simulink model "TestHiTechnicColorSensor"  (Simulink 6.4)
settings: Solver=FixedStepDiscrete  SolverMode=SingleTasking  StartTime=0  StopTime=inf  FixedStep=0.001  RelTol=1e-3
libraries: simulink x9, ecrobot_nxt_lib x8
settings Model: Creator=tchikama  LastModifiedBy=tchikama  ProdHWDeviceType=ARM7
settings DataIOCC: SaveOutput=off  SignalLogging=off  SaveTime=off
settings OptimizationCC: InlineParams=on  InlineInvariantSignals=on  RollThreshold=2  StateBitsets=on  DataBitsets=on  UseTempVars=on  InitFltsAndDblsToZero=off  NoFixptDivByZeroProtection=on  EfficientFloat2IntCast=on  OptimizeModelRefInitCode=on  LifeSpan=1
settings DebuggingCC: ConsistencyChecking=warning  SignalInfNanChecking=warning  ReadBeforeWriteMsg=DisableAll  WriteAfterWriteMsg=DisableAll  WriteAfterReadMsg=DisableAll  AlgebraicLoopMsg=error  CheckExecutionContextPreStartOutputMsg=on  CheckExecutionContextRuntimeOutputMsg=on  SolverPrmCheckMsg=none  SingleTaskRateTransMsg=warning  TasksWithSamePriorityMsg=none  IntegerOverflowMsg=error  ParameterPrecisionLossMsg=none  UnconnectedInputMsg=error  UnconnectedOutputMsg=error  UnconnectedLineMsg=error  UniqueDataStoreMsg=error  BusObjectLabelMismatch=error  RootOutportRequireBusObject=error  ModelReferenceIOMsg=warning  ModelReferenceVersionMismatchMessage=warning  ModelReferenceIOMismatchMessage=warning
settings HardwareCC: ProdIntDivRoundTo=Zero  ProdEndianess=LittleEndian  ProdHWDeviceType=ARM7  TargetHWDeviceType=32-bit Generic
settings ModelReferenceCC: ModelReferenceNumInstancesAllowed=Single
settings RTWCC: SystemTargetFile=ert.tlc  GenCodeOnly=on  GenerateMakefile=off  TemplateMakefile=ert_default_tmf  Description=Real-Time Workshop Embedded Coder (no auto configuration)  GenerateReport=on  RTWVerbose=off  ProcessScript=ert_make_rtw_hook  IncludeHyperlinkInReport=on  LaunchReport=on
settings CodeAppCC: ForceParamTrailComments=on  IgnoreCustomStorageClasses=off  SFDataObjDesc=on  PrefixModelToSubsysFcnNames=off  CustomSymbolStrGlobalVar=rt$N$M  CustomSymbolStrType=$N$M  CustomSymbolStrFcn=$N$M$F  CustomSymbolStrMacro=$N$M  InsertBlockDesc=on
settings ERTTargetCC: TargetFcnLib=ansi_tfl_tmw.mat  GenFloatMathFcnCalls=GNU  IncludeMdlTerminateFcn=off  SuppressErrorStatus=on  IncludeERTFirstTime=on  SupportAbsoluteTime=off  SupportNonFinite=off  SupportComplex=off  PurelyIntegerCode=on  InlinedParameterPlacement=NonHierarchical  RootIOFormat=Structure reference  ERTCustomFileTemplate=example_file_process.tlc  InitialValueSource=Model

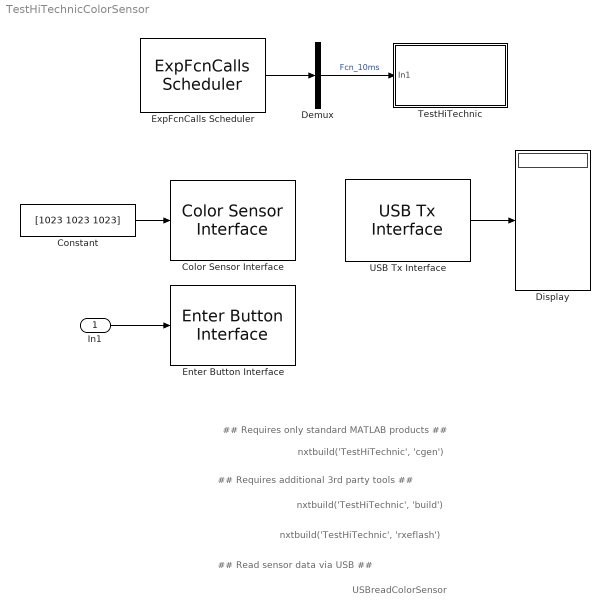
== system TestHiTechnicColorSensor ==
  note: nxtbuild('TestHiTechnic', 'build')
  note: nxtbuild('TestHiTechnic', 'rxeflash')
  note: nxtbuild('TestHiTechnic', 'cgen')
  note: ## Requires only standard MATLAB products ##
  note: ## Requires additional 3rd party tools ##
  note: ## Read sensor data via USB ##
  note: USBreadColorSensor
  In1 : Inport
  Color Sensor Interface : ecrobot_nxt_lib/Color Sensor Interface  SystemSampleTime=-1  ip=S1
  Constant : Constant  Value=[1023 1023 1023]  OutDataType=sfix(16)  ConRadixGroup=Use specified scaling  OutScaling=2^0  SampleTime=inf  FramePeriod=inf
  Demux : Demux  Outputs=1
  Display : Display
  Enter Button Interface : ecrobot_nxt_lib/Enter Button Interface  SystemSampleTime=-1
  ExpFcnCalls Scheduler : ecrobot_nxt_lib/ExpFcnCalls Scheduler  fcname='Fcn_10ms'  fctrigger=[10]  ts=0.001  platform=OSEK  stacksize=[512]  bd_mode=Slave
  TestHiTechnic : Subsystem
  USB Tx Interface : ecrobot_nxt_lib/USB Tx Interface  SystemSampleTime=-1
  wires:
  ExpFcnCalls Scheduler/1 -> Demux/1
  Demux/1 -> TestHiTechnic/1(In1)  "Fcn_10ms"
  Constant/1 -> Color Sensor Interface/1
  USB Tx Interface/1 -> Display/1
  In1/1 -> Enter Button Interface/1

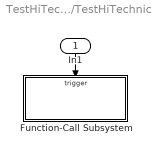
== system TestHiTechnicColorSensor/TestHiTechnic ==
  In1 : Inport  Orientation=down
  Function-Call Subsystem : Subsystem  TreatAsAtomicUnit=on
  wires:
  In1/1 -> Function-Call Subsystem/Trigger

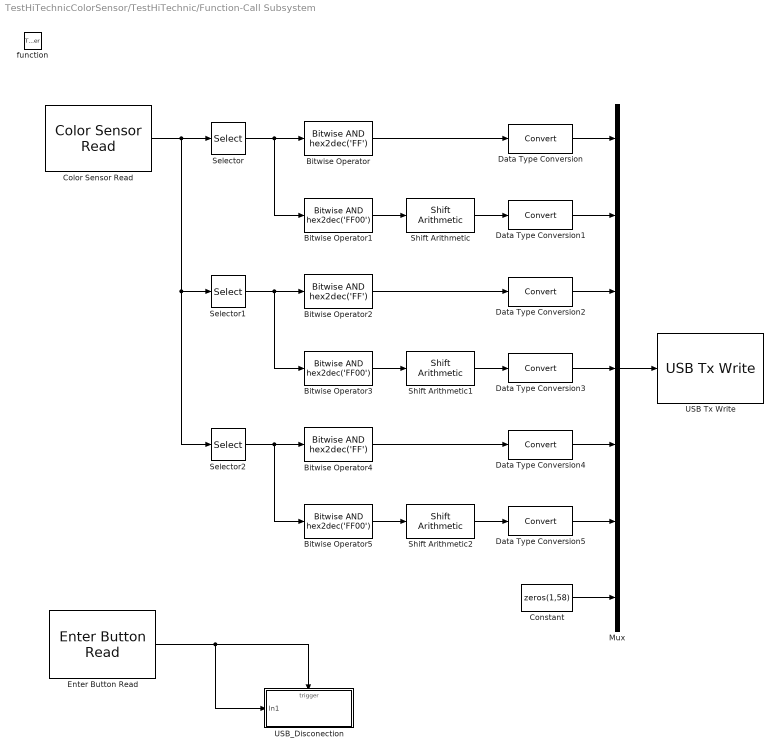
== system TestHiTechnicColorSensor/TestHiTechnic/Function-Call Subsystem ==
  function : TriggerPort  TriggerType=function-call
  Bitwise Operator : simulink/Logic and Bit Operations/Bitwise Operator  logicop=AND  UseBitMask=on  BitMask=hex2dec('FF')  BitMaskRealWorld=Stored Integer
  Bitwise Operator1 : simulink/Logic and Bit Operations/Bitwise Operator  logicop=AND  UseBitMask=on  BitMask=hex2dec('FF00')  BitMaskRealWorld=Stored Integer
  Bitwise Operator2 : simulink/Logic and Bit Operations/Bitwise Operator  logicop=AND  UseBitMask=on  BitMask=hex2dec('FF')  BitMaskRealWorld=Stored Integer
  Bitwise Operator3 : simulink/Logic and Bit Operations/Bitwise Operator  logicop=AND  UseBitMask=on  BitMask=hex2dec('FF00')  BitMaskRealWorld=Stored Integer
  Bitwise Operator4 : simulink/Logic and Bit Operations/Bitwise Operator  logicop=AND  UseBitMask=on  BitMask=hex2dec('FF')  BitMaskRealWorld=Stored Integer
  Bitwise Operator5 : simulink/Logic and Bit Operations/Bitwise Operator  logicop=AND  UseBitMask=on  BitMask=hex2dec('FF00')  BitMaskRealWorld=Stored Integer
  Color Sensor Read : ecrobot_nxt_lib/Color Sensor Read  ip=S1
  Constant : Constant  Value=zeros(1,58)  OutDataTypeMode=uint8  OutDataType=sfix(16)  ConRadixGroup=Use specified scaling  OutScaling=2^0  SampleTime=inf  FramePeriod=inf
  Data Type Conversion{,1..5} (6 alike) : DataTypeConversion  OutDataTypeMode=uint8
  Enter Button Read : ecrobot_nxt_lib/Enter Button Read  SystemSampleTime=-1
  Mux : Mux  Inputs=7
  Selector : Selector  Elements=[1]  InputPortWidth=3
  Selector1 : Selector  Elements=[2]  InputPortWidth=3
  Selector2 : Selector  Elements=[3]  InputPortWidth=3
  Shift Arithmetic : simulink/Logic and Bit Operations/Shift Arithmetic  SystemSampleTime=-1  nBitShiftRight=8  nBinPtShiftRight=0
  Shift Arithmetic1 : simulink/Logic and Bit Operations/Shift Arithmetic  SystemSampleTime=-1  nBitShiftRight=8  nBinPtShiftRight=0
  Shift Arithmetic2 : simulink/Logic and Bit Operations/Shift Arithmetic  SystemSampleTime=-1  nBitShiftRight=8  nBinPtShiftRight=0
  USB Tx Write : ecrobot_nxt_lib/USB Tx Write
  USB_Disconection : Subsystem  TreatAsAtomicUnit=on
  wires:
  Data Type Conversion/1 -> Mux/1
  Mux/1 -> USB Tx Write/1
  Color Sensor Read/1 -> Selector/1, Selector1/1, Selector2/1
  Selector/1 -> Bitwise Operator/1, Bitwise Operator1/1
  Bitwise Operator/1 -> Data Type Conversion/1
  Constant/1 -> Mux/7
  Bitwise Operator1/1 -> Shift Arithmetic/1
  Data Type Conversion1/1 -> Mux/2
  Data Type Conversion2/1 -> Mux/3
  Selector1/1 -> Bitwise Operator2/1, Bitwise Operator3/1
  Bitwise Operator2/1 -> Data Type Conversion2/1
  Bitwise Operator3/1 -> Shift Arithmetic1/1
  Data Type Conversion3/1 -> Mux/4
  Data Type Conversion4/1 -> Mux/5
  Selector2/1 -> Bitwise Operator4/1, Bitwise Operator5/1
  Bitwise Operator4/1 -> Data Type Conversion4/1
  Bitwise Operator5/1 -> Shift Arithmetic2/1
  Data Type Conversion5/1 -> Mux/6
  Shift Arithmetic/1 -> Data Type Conversion1/1
  Shift Arithmetic1/1 -> Data Type Conversion3/1
  Shift Arithmetic2/1 -> Data Type Conversion5/1
  Enter Button Read/1 -> USB_Disconection/Trigger, USB_Disconection/1(In1)

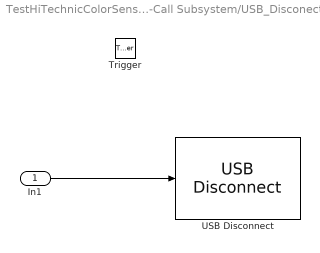
== system TestHiTechnicColorSensor/TestHiTechnic/Function-Call Subsystem/USB_Disconection ==
  In1 : Inport
  Trigger : TriggerPort
  USB Disconnect : ecrobot_nxt_lib/USB Disconnect
  wires:
  In1/1 -> USB Disconnect/1
